simulink model "DynamicsPID_CompleteTest"  (R2018b)
settings: Solver=ode5  StartTime=0.0  StopTime=10  FixedStep=0.0001  RelTol=1e-3
PreLoadFcn:
  | load('Arm6SimscapeData.mat');
model workspace: external: MAT-File E:\SixRobotArm\Simscape_Simulation\Arm6SimscapeData.mat (data not in the file)
values from neighbouring files (symbols this model uses):
  smiData =     [Arm6SimscapeData.mat]
undefined symbols (not defined in the file or in its folder): X, Y, Z
libraries: sm_lib x36, nesl_utility x31, fl_lib x13, simulink x6
(part 1 of 2)
settings Model: SimulationMode=accelerator  Creator=Administrator  LastModifiedBy=Jeason
settings SolverCC: AutoInsertRateTranBlk=on
settings DataIOCC: ReturnWorkspaceOutputs=on
settings ExplorerConfigSet: InternalSimMechanicsExplorerSettings="<ExplorerConfiguration><canonicalview>planar_xy</canonicalview><AnimationSetting><BasePlaybackSpeed>1.0</BasePlaybackSpeed><PlaybackSpeedFactor>1.0</PlaybackSpeedFactor></AnimationSetting><TilePanel><TileInfo><Tiles Columns=\"1\" Count=\"1\" Rows=\"1\"><Column Weight=\"1\"/><Row Weight=\"1\"/><Tile Height=\"1\" Width=\"1\" X=\"0\" Y=\"0\"/></Tiles></TileInfo><SceneInfo><SceneViewer><BGColor><R>0.60000002384185791</R><G>0.60000002384185791</G><B>0.60000002384185791</B></BGColor><Camera><DoPerspective>off</DoPerspective><Position><X>0.529425685588477024</X><Y>0.96968881474758839</Y><Z>0.531520526083879341</Z></Position><Center><X>-0.0479245836011489429</X><Y>0.392338545557962604</Y><Z>-0.0458297431057466537</Z></Center><Up><X>-0.408248290463863073</X><Y>0.816496580927726145</Y><Z>-0.408248290463863073</Z></Up><ViewLimDist>1</ViewLimDist><YLim>0.78131541566616991</YLim><XLim>0.557104420151891211</XLim></Camera></SceneViewer></SceneInfo></TilePanel><MechEditorPanel><Cameras/><GfxPanelCameraMap/><VideoCreator><PlaybackSpeedRatio>1.0</PlaybackSpeedRatio><FrameRate>30</FrameRate><VideoFormat>MPEG-4</VideoFormat><FrameSize>[400 400]</FrameSize></VideoCreator></MechEditorPanel></ExplorerConfiguration>"

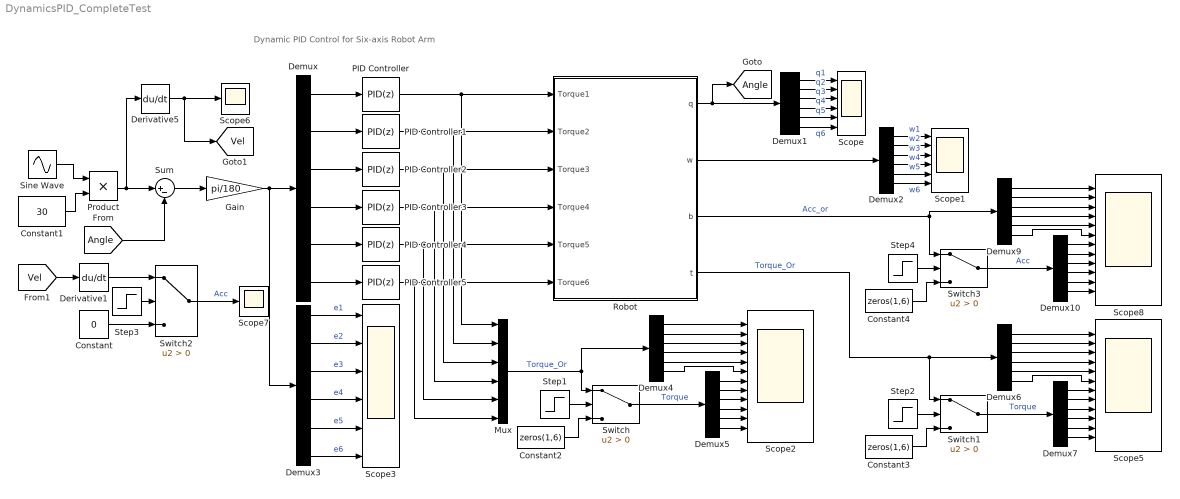
== system DynamicsPID_CompleteTest ==
  note: Dynamic PID Control for Six-axis Robot Arm
  Constant : Constant  Value=0
  Constant1 : Constant  Value=30
  Constant2 : Constant  Value=zeros(1,6)
  Constant3 : Constant  Value=zeros(1,6)
  Constant4 : Constant  Value=zeros(1,6)
  Demux{,1..7,9..10} (10 alike) : Demux  Outputs=6
  Derivative1 : Derivative
  Derivative5 : Derivative
  Gain : Gain  Gain=pi/180
  Mux : Mux  Inputs=6
  PID Controller : simulink/Continuous/PID Controller  Controller=PID  Form=Parallel  TimeDomain=Discrete-time  SampleTime=-1  IntegratorMethod=Forward Euler  FilterMethod=Forward Euler  ControllerParametersSource=internal  P=6578.50187258326  I=281577.896683485  D=27.3665494202085  UseFilter=on  N=17023.3251187192  TunerSelectOption=Transfer Function Based (PID Tuner App)  InitialConditionSource=internal  InitialConditionForIntegrator=0  InitialConditionForFilter=0  DifferentiatorICPrevScaledInput=0  ExternalReset=none  TrackingMode=off  Kt=1  LimitOutput=off  UpperSaturationLimit=inf  LowerSaturationLimit=-inf  LinearizeAsGain=on  AntiWindupMode=none  Kb=1  POutMin=[]  POutMax=[]  IOutMin=[]  IOutMax=[]  DOutMin=[]  DOutMax=[]  NOutMin=[]  NOutMax=[]  SumOutMin=[]  SumOutMax=[]  SaturationOutMin=[]  SaturationOutMax=[]  PParamMin=[]  PParamMax=[]  IParamMin=[]  IParamMax=[]  DParamMin=[]  DParamMax=[]  NParamMin=[]  NParamMax=[]  KbParamMin=[]  KbParamMax=[]  KtParamMin=[]  KtParamMax=[]  KbOutMin=[]  KbOutMax=[]  KtOutMin=[]  KtOutMax=[]  IntegratorOutMin=[]  IntegratorOutMax=[]  FilterOutMin=[]  FilterOutMax=[]  SumI1OutMin=[]  SumI1OutMax=[]  SumI2OutMin=[]  SumI2OutMax=[]  SumI3OutMin=[]  SumI3OutMax=[]  SumI4OutMin=[]  SumI4OutMax=[]  SumDOutMin=[]  SumDOutMax=[]  DifferentiatorOutMin=[]  DifferentiatorOutMax=[]  FilterDiffOutCoefMin=[]  FilterDiffOutCoefMax=[]  ReciprocalOutMin=[]  ReciprocalOutMax=[]  SumDenOutMin=[]  SumDenOutMax=[]  SumNumOutMin=[]  SumNumOutMax=[]  DivideOutMin=[]  DivideOutMax=[]  IntegratorContinuousStateAttributes=''  IntegratorStateMustResolveToSignalObject=off  IntegratorRTWStateStorageClass=Auto  FilterContinuousStateAttributes=''  FilterStateMustResolveToSignalObject=off  FilterRTWStateStorageClass=Auto  ParallelPVariant=InternalParameters  IdealPVariant=Disabled  IVariant=InternalParameters  DVariant=InternalParameters  IntegratorVariant=Discrete  SatVariant=Disabled  AWVariant=Passthrough  PCopyVariant=Disabled  TRVariant=Disabled  FdbkBlocksVariant=Forward  IdealPFdbkVariant=Disabled  SatFdbkVariant=Disabled  DerivativeFilterVariant=ForwardEulerFilter  NVariant=InternalParameters  NCopyVariant=Disabled  FilterICVariant=InternalICsFilter  IntegratorICVariant=InternalICs  ExternalResetVariant=Disabled  TRSumVariant=Passthrough  SumFdbkVariant=Disabled  SumVariant=Sum_PID
  PID Controller1 : simulink/Continuous/PID Controller  Controller=PID  Form=Parallel  TimeDomain=Discrete-time  SampleTime=-1  IntegratorMethod=Forward Euler  FilterMethod=Forward Euler  ControllerParametersSource=internal  P=10668.8664662437  I=445184.60715373  D=63.0054233348583  UseFilter=on  N=6162.16152893693  TunerSelectOption=Transfer Function Based (PID Tuner App)  InitialConditionSource=internal  InitialConditionForIntegrator=0  InitialConditionForFilter=0  DifferentiatorICPrevScaledInput=0  ExternalReset=none  TrackingMode=off  Kt=1  LimitOutput=off  UpperSaturationLimit=inf  LowerSaturationLimit=-inf  LinearizeAsGain=on  AntiWindupMode=none  Kb=1  POutMin=[]  POutMax=[]  IOutMin=[]  IOutMax=[]  DOutMin=[]  DOutMax=[]  NOutMin=[]  NOutMax=[]  SumOutMin=[]  SumOutMax=[]  SaturationOutMin=[]  SaturationOutMax=[]  PParamMin=[]  PParamMax=[]  IParamMin=[]  IParamMax=[]  DParamMin=[]  DParamMax=[]  NParamMin=[]  NParamMax=[]  KbParamMin=[]  KbParamMax=[]  KtParamMin=[]  KtParamMax=[]  KbOutMin=[]  KbOutMax=[]  KtOutMin=[]  KtOutMax=[]  IntegratorOutMin=[]  IntegratorOutMax=[]  FilterOutMin=[]  FilterOutMax=[]  SumI1OutMin=[]  SumI1OutMax=[]  SumI2OutMin=[]  SumI2OutMax=[]  SumI3OutMin=[]  SumI3OutMax=[]  SumI4OutMin=[]  SumI4OutMax=[]  SumDOutMin=[]  SumDOutMax=[]  DifferentiatorOutMin=[]  DifferentiatorOutMax=[]  FilterDiffOutCoefMin=[]  FilterDiffOutCoefMax=[]  ReciprocalOutMin=[]  ReciprocalOutMax=[]  SumDenOutMin=[]  SumDenOutMax=[]  SumNumOutMin=[]  SumNumOutMax=[]  DivideOutMin=[]  DivideOutMax=[]  IntegratorContinuousStateAttributes=''  IntegratorStateMustResolveToSignalObject=off  IntegratorRTWStateStorageClass=Auto  FilterContinuousStateAttributes=''  FilterStateMustResolveToSignalObject=off  FilterRTWStateStorageClass=Auto  ParallelPVariant=InternalParameters  IdealPVariant=Disabled  IVariant=InternalParameters  DVariant=InternalParameters  IntegratorVariant=Discrete  SatVariant=Disabled  AWVariant=Passthrough  PCopyVariant=Disabled  TRVariant=Disabled  FdbkBlocksVariant=Forward  IdealPFdbkVariant=Disabled  SatFdbkVariant=Disabled  DerivativeFilterVariant=ForwardEulerFilter  NVariant=InternalParameters  NCopyVariant=Disabled  FilterICVariant=InternalICsFilter  IntegratorICVariant=InternalICs  ExternalResetVariant=Disabled  TRSumVariant=Passthrough  SumFdbkVariant=Disabled  SumVariant=Sum_PID
  PID Controller2 : simulink/Continuous/PID Controller  Controller=PID  Form=Parallel  TimeDomain=Discrete-time  SampleTime=-1  IntegratorMethod=Forward Euler  FilterMethod=Forward Euler  ControllerParametersSource=internal  P=13614.8176617989  I=1609883.93215342  D=16.7397300352701  UseFilter=on  N=18647.3427476524  TunerSelectOption=Transfer Function Based (PID Tuner App)  InitialConditionSource=internal  InitialConditionForIntegrator=0  InitialConditionForFilter=0  DifferentiatorICPrevScaledInput=0  ExternalReset=none  TrackingMode=off  Kt=1  LimitOutput=off  UpperSaturationLimit=inf  LowerSaturationLimit=-inf  LinearizeAsGain=on  AntiWindupMode=none  Kb=1  POutMin=[]  POutMax=[]  IOutMin=[]  IOutMax=[]  DOutMin=[]  DOutMax=[]  NOutMin=[]  NOutMax=[]  SumOutMin=[]  SumOutMax=[]  SaturationOutMin=[]  SaturationOutMax=[]  PParamMin=[]  PParamMax=[]  IParamMin=[]  IParamMax=[]  DParamMin=[]  DParamMax=[]  NParamMin=[]  NParamMax=[]  KbParamMin=[]  KbParamMax=[]  KtParamMin=[]  KtParamMax=[]  KbOutMin=[]  KbOutMax=[]  KtOutMin=[]  KtOutMax=[]  IntegratorOutMin=[]  IntegratorOutMax=[]  FilterOutMin=[]  FilterOutMax=[]  SumI1OutMin=[]  SumI1OutMax=[]  SumI2OutMin=[]  SumI2OutMax=[]  SumI3OutMin=[]  SumI3OutMax=[]  SumI4OutMin=[]  SumI4OutMax=[]  SumDOutMin=[]  SumDOutMax=[]  DifferentiatorOutMin=[]  DifferentiatorOutMax=[]  FilterDiffOutCoefMin=[]  FilterDiffOutCoefMax=[]  ReciprocalOutMin=[]  ReciprocalOutMax=[]  SumDenOutMin=[]  SumDenOutMax=[]  SumNumOutMin=[]  SumNumOutMax=[]  DivideOutMin=[]  DivideOutMax=[]  IntegratorContinuousStateAttributes=''  IntegratorStateMustResolveToSignalObject=off  IntegratorRTWStateStorageClass=Auto  FilterContinuousStateAttributes=''  FilterStateMustResolveToSignalObject=off  FilterRTWStateStorageClass=Auto  ParallelPVariant=InternalParameters  IdealPVariant=Disabled  IVariant=InternalParameters  DVariant=InternalParameters  IntegratorVariant=Discrete  SatVariant=Disabled  AWVariant=Passthrough  PCopyVariant=Disabled  TRVariant=Disabled  FdbkBlocksVariant=Forward  IdealPFdbkVariant=Disabled  SatFdbkVariant=Disabled  DerivativeFilterVariant=ForwardEulerFilter  NVariant=InternalParameters  NCopyVariant=Disabled  FilterICVariant=InternalICsFilter  IntegratorICVariant=InternalICs  ExternalResetVariant=Disabled  TRSumVariant=Passthrough  SumFdbkVariant=Disabled  SumVariant=Sum_PID
  PID Controller3 : simulink/Continuous/PID Controller  Controller=PID  Form=Parallel  TimeDomain=Discrete-time  SampleTime=-1  IntegratorMethod=Forward Euler  FilterMethod=Forward Euler  ControllerParametersSource=internal  P=2278.44727281027  I=57632.5068461777  D=4.78900982736188  UseFilter=on  N=12334.3834454525  TunerSelectOption=Transfer Function Based (PID Tuner App)  InitialConditionSource=internal  InitialConditionForIntegrator=0  InitialConditionForFilter=0  DifferentiatorICPrevScaledInput=0  ExternalReset=none  TrackingMode=off  Kt=1  LimitOutput=off  UpperSaturationLimit=inf  LowerSaturationLimit=-inf  LinearizeAsGain=on  AntiWindupMode=none  Kb=1  POutMin=[]  POutMax=[]  IOutMin=[]  IOutMax=[]  DOutMin=[]  DOutMax=[]  NOutMin=[]  NOutMax=[]  SumOutMin=[]  SumOutMax=[]  SaturationOutMin=[]  SaturationOutMax=[]  PParamMin=[]  PParamMax=[]  IParamMin=[]  IParamMax=[]  DParamMin=[]  DParamMax=[]  NParamMin=[]  NParamMax=[]  KbParamMin=[]  KbParamMax=[]  KtParamMin=[]  KtParamMax=[]  KbOutMin=[]  KbOutMax=[]  KtOutMin=[]  KtOutMax=[]  IntegratorOutMin=[]  IntegratorOutMax=[]  FilterOutMin=[]  FilterOutMax=[]  SumI1OutMin=[]  SumI1OutMax=[]  SumI2OutMin=[]  SumI2OutMax=[]  SumI3OutMin=[]  SumI3OutMax=[]  SumI4OutMin=[]  SumI4OutMax=[]  SumDOutMin=[]  SumDOutMax=[]  DifferentiatorOutMin=[]  DifferentiatorOutMax=[]  FilterDiffOutCoefMin=[]  FilterDiffOutCoefMax=[]  ReciprocalOutMin=[]  ReciprocalOutMax=[]  SumDenOutMin=[]  SumDenOutMax=[]  SumNumOutMin=[]  SumNumOutMax=[]  DivideOutMin=[]  DivideOutMax=[]  IntegratorContinuousStateAttributes=''  IntegratorStateMustResolveToSignalObject=off  IntegratorRTWStateStorageClass=Auto  FilterContinuousStateAttributes=''  FilterStateMustResolveToSignalObject=off  FilterRTWStateStorageClass=Auto  ParallelPVariant=InternalParameters  IdealPVariant=Disabled  IVariant=InternalParameters  DVariant=InternalParameters  IntegratorVariant=Discrete  SatVariant=Disabled  AWVariant=Passthrough  PCopyVariant=Disabled  TRVariant=Disabled  FdbkBlocksVariant=Forward  IdealPFdbkVariant=Disabled  SatFdbkVariant=Disabled  DerivativeFilterVariant=ForwardEulerFilter  NVariant=InternalParameters  NCopyVariant=Disabled  FilterICVariant=InternalICsFilter  IntegratorICVariant=InternalICs  ExternalResetVariant=Disabled  TRSumVariant=Passthrough  SumFdbkVariant=Disabled  SumVariant=Sum_PID
  PID Controller4 : simulink/Continuous/PID Controller  Controller=PID  Form=Parallel  TimeDomain=Discrete-time  SampleTime=-1  IntegratorMethod=Forward Euler  FilterMethod=Forward Euler  ControllerParametersSource=internal  P=162.012170441032  I=2991.2299773876  D=1.94609590633376  UseFilter=on  N=18952.9125503668  TunerSelectOption=Transfer Function Based (PID Tuner App)  InitialConditionSource=internal  InitialConditionForIntegrator=0  InitialConditionForFilter=0  DifferentiatorICPrevScaledInput=0  ExternalReset=none  TrackingMode=off  Kt=1  LimitOutput=off  UpperSaturationLimit=inf  LowerSaturationLimit=-inf  LinearizeAsGain=on  AntiWindupMode=none  Kb=1  POutMin=[]  POutMax=[]  IOutMin=[]  IOutMax=[]  DOutMin=[]  DOutMax=[]  NOutMin=[]  NOutMax=[]  SumOutMin=[]  SumOutMax=[]  SaturationOutMin=[]  SaturationOutMax=[]  PParamMin=[]  PParamMax=[]  IParamMin=[]  IParamMax=[]  DParamMin=[]  DParamMax=[]  NParamMin=[]  NParamMax=[]  KbParamMin=[]  KbParamMax=[]  KtParamMin=[]  KtParamMax=[]  KbOutMin=[]  KbOutMax=[]  KtOutMin=[]  KtOutMax=[]  IntegratorOutMin=[]  IntegratorOutMax=[]  FilterOutMin=[]  FilterOutMax=[]  SumI1OutMin=[]  SumI1OutMax=[]  SumI2OutMin=[]  SumI2OutMax=[]  SumI3OutMin=[]  SumI3OutMax=[]  SumI4OutMin=[]  SumI4OutMax=[]  SumDOutMin=[]  SumDOutMax=[]  DifferentiatorOutMin=[]  DifferentiatorOutMax=[]  FilterDiffOutCoefMin=[]  FilterDiffOutCoefMax=[]  ReciprocalOutMin=[]  ReciprocalOutMax=[]  SumDenOutMin=[]  SumDenOutMax=[]  SumNumOutMin=[]  SumNumOutMax=[]  DivideOutMin=[]  DivideOutMax=[]  IntegratorContinuousStateAttributes=''  IntegratorStateMustResolveToSignalObject=off  IntegratorRTWStateStorageClass=Auto  FilterContinuousStateAttributes=''  FilterStateMustResolveToSignalObject=off  FilterRTWStateStorageClass=Auto  ParallelPVariant=InternalParameters  IdealPVariant=Disabled  IVariant=InternalParameters  DVariant=InternalParameters  IntegratorVariant=Discrete  SatVariant=Disabled  AWVariant=Passthrough  PCopyVariant=Disabled  TRVariant=Disabled  FdbkBlocksVariant=Forward  IdealPFdbkVariant=Disabled  SatFdbkVariant=Disabled  DerivativeFilterVariant=ForwardEulerFilter  NVariant=InternalParameters  NCopyVariant=Disabled  FilterICVariant=InternalICsFilter  IntegratorICVariant=InternalICs  ExternalResetVariant=Disabled  TRSumVariant=Passthrough  SumFdbkVariant=Disabled  SumVariant=Sum_PID
  PID Controller5 : simulink/Continuous/PID Controller  Controller=PID  Form=Parallel  TimeDomain=Discrete-time  SampleTime=-1  IntegratorMethod=Forward Euler  FilterMethod=Forward Euler  ControllerParametersSource=internal  P=53.1250888383144  I=2127.20939788441  D=0.32148544609688  UseFilter=on  N=3458.79738025908  TunerSelectOption=Transfer Function Based (PID Tuner App)  InitialConditionSource=internal  InitialConditionForIntegrator=0  InitialConditionForFilter=0  DifferentiatorICPrevScaledInput=0  ExternalReset=none  TrackingMode=off  Kt=1  LimitOutput=off  UpperSaturationLimit=inf  LowerSaturationLimit=-inf  LinearizeAsGain=on  AntiWindupMode=none  Kb=1  POutMin=[]  POutMax=[]  IOutMin=[]  IOutMax=[]  DOutMin=[]  DOutMax=[]  NOutMin=[]  NOutMax=[]  SumOutMin=[]  SumOutMax=[]  SaturationOutMin=[]  SaturationOutMax=[]  PParamMin=[]  PParamMax=[]  IParamMin=[]  IParamMax=[]  DParamMin=[]  DParamMax=[]  NParamMin=[]  NParamMax=[]  KbParamMin=[]  KbParamMax=[]  KtParamMin=[]  KtParamMax=[]  KbOutMin=[]  KbOutMax=[]  KtOutMin=[]  KtOutMax=[]  IntegratorOutMin=[]  IntegratorOutMax=[]  FilterOutMin=[]  FilterOutMax=[]  SumI1OutMin=[]  SumI1OutMax=[]  SumI2OutMin=[]  SumI2OutMax=[]  SumI3OutMin=[]  SumI3OutMax=[]  SumI4OutMin=[]  SumI4OutMax=[]  SumDOutMin=[]  SumDOutMax=[]  DifferentiatorOutMin=[]  DifferentiatorOutMax=[]  FilterDiffOutCoefMin=[]  FilterDiffOutCoefMax=[]  ReciprocalOutMin=[]  ReciprocalOutMax=[]  SumDenOutMin=[]  SumDenOutMax=[]  SumNumOutMin=[]  SumNumOutMax=[]  DivideOutMin=[]  DivideOutMax=[]  IntegratorContinuousStateAttributes=''  IntegratorStateMustResolveToSignalObject=off  IntegratorRTWStateStorageClass=Auto  FilterContinuousStateAttributes=''  FilterStateMustResolveToSignalObject=off  FilterRTWStateStorageClass=Auto  ParallelPVariant=InternalParameters  IdealPVariant=Disabled  IVariant=InternalParameters  DVariant=InternalParameters  IntegratorVariant=Discrete  SatVariant=Disabled  AWVariant=Passthrough  PCopyVariant=Disabled  TRVariant=Disabled  FdbkBlocksVariant=Forward  IdealPFdbkVariant=Disabled  SatFdbkVariant=Disabled  DerivativeFilterVariant=ForwardEulerFilter  NVariant=InternalParameters  NCopyVariant=Disabled  FilterICVariant=InternalICsFilter  IntegratorICVariant=InternalICs  ExternalResetVariant=Disabled  TRSumVariant=Passthrough  SumFdbkVariant=Disabled  SumVariant=Sum_PID
  Product : Product
  Robot : Subsystem
  Scope : Scope  NumInputPorts=6
  Scope1 : Scope  NumInputPorts=6
  Scope2 : Scope  NumInputPorts=12
  Scope3 : Scope  NumInputPorts=6
  Scope5 : Scope  NumInputPorts=12
  Scope6 : Scope
  Scope7 : Scope
  Scope8 : Scope  NumInputPorts=12
  Sine Wave : Sin  Frequency=0.25*2*pi
  Step1 : Step  Time=0.3  After=2
  Step2 : Step  Time=0.1  After=2
  Step3 : Step  Time=0.1  After=2
  Step4 : Step  Time=0.3  After=2
  Sum : Sum  Inputs=|+-
  Switch{,1..3} (4 alike) : Switch  Criteria=u2 > Threshold
  tag scope: Angle=global, Vel=global
  wires:
  Robot/1(q) -> Demux1/1, [Angle]
  Demux1/1 -> Scope/1  "q1"
  Demux1/2 -> Scope/2  "q2"
  Demux1/3 -> Scope/3  "q3"
  Demux1/4 -> Scope/4  "q4"
  Demux1/5 -> Scope/5  "q5"
  Demux1/6 -> Scope/6  "q6"
  Robot/2(w) -> Demux2/1
  Demux2/1 -> Scope1/1  "w1"
  Demux2/2 -> Scope1/2  "w2"
  Demux2/3 -> Scope1/3  "w3"
  Demux2/4 -> Scope1/4  "w4"
  Demux2/5 -> Scope1/5  "w5"
  Demux2/6 -> Scope1/6  "w6"
  Constant1/1 -> Product/2
  Sine Wave/1 -> Product/1
  Constant2/1 -> Switch/3
  Step1/1 -> Switch/2
  Mux/1 -> Switch/1, Demux4/1  "Torque_Or"
  Sum/1 -> Gain/1
  [Angle] -> Sum/2
  Gain/1 -> Demux3/1, Demux/1
  Demux/1 -> PID Controller/1
  Demux/2 -> PID Controller1/1
  Demux/3 -> PID Controller2/1
  Demux/4 -> PID Controller3/1
  Demux/5 -> PID Controller4/1
  Demux/6 -> PID Controller5/1
  PID Controller/1 -> Robot/1(Torque1), Mux/1
  PID Controller1/1 -> Robot/2(Torque2), Mux/2
  PID Controller2/1 -> Robot/3(Torque3), Mux/3
  PID Controller3/1 -> Robot/4(Torque4), Mux/4
  PID Controller4/1 -> Robot/5(Torque5), Mux/5
  PID Controller5/1 -> Robot/6(Torque6), Mux/6
  Demux3/1 -> Scope3/1  "e1"
  Demux3/2 -> Scope3/2  "e2"
  Demux3/3 -> Scope3/3  "e3"
  Demux3/4 -> Scope3/4  "e4"
  Demux3/5 -> Scope3/5  "e5"
  Demux3/6 -> Scope3/6  "e6"
  Demux4/2 -> Scope2/2
  Demux4/1 -> Scope2/1
  Demux4/3 -> Scope2/3
  Demux4/4 -> Scope2/4
  Demux4/5 -> Scope2/5
  Demux4/6 -> Scope2/6
  Demux5/2 -> Scope2/8
  Demux5/1 -> Scope2/7
  Demux5/3 -> Scope2/9
  Demux5/4 -> Scope2/10
  Demux5/5 -> Scope2/11
  Demux5/6 -> Scope2/12
  Switch/1 -> Demux5/1  "Torque"
  Switch1/1 -> Demux7/1  "Torque"
  Demux7/6 -> Scope5/12
  Demux7/5 -> Scope5/11
  Demux7/4 -> Scope5/10
  Demux7/3 -> Scope5/9
  Demux7/1 -> Scope5/7
  Demux7/2 -> Scope5/8
  Demux6/6 -> Scope5/6
  Demux6/5 -> Scope5/5
  Demux6/4 -> Scope5/4
  Demux6/3 -> Scope5/3
  Demux6/1 -> Scope5/1
  Demux6/2 -> Scope5/2
  Robot/4(t) -> Switch1/1, Demux6/1  "Torque_Or"
  Step2/1 -> Switch1/2
  Constant3/1 -> Switch1/3
  Product/1 -> Sum/1, Derivative5/1
  Derivative5/1 -> [Vel], Scope6/1
  Derivative1/1 -> Switch2/1
  Step3/1 -> Switch2/2
  [Vel] -> Derivative1/1
  Constant/1 -> Switch2/3
  Switch2/1 -> Scope7/1  "Acc"
  Constant4/1 -> Switch3/3
  Step4/1 -> Switch3/2
  Robot/3(b) -> Demux9/1, Switch3/1  "Acc_or"
  Demux9/2 -> Scope8/2
  Demux9/1 -> Scope8/1
  Demux9/3 -> Scope8/3
  Demux9/4 -> Scope8/4
  Demux9/5 -> Scope8/5
  Demux9/6 -> Scope8/6
  Demux10/2 -> Scope8/8
  Demux10/1 -> Scope8/7
  Demux10/3 -> Scope8/9
  Demux10/4 -> Scope8/10
  Demux10/5 -> Scope8/11
  Demux10/6 -> Scope8/12
  Switch3/1 -> Demux10/1  "Acc"

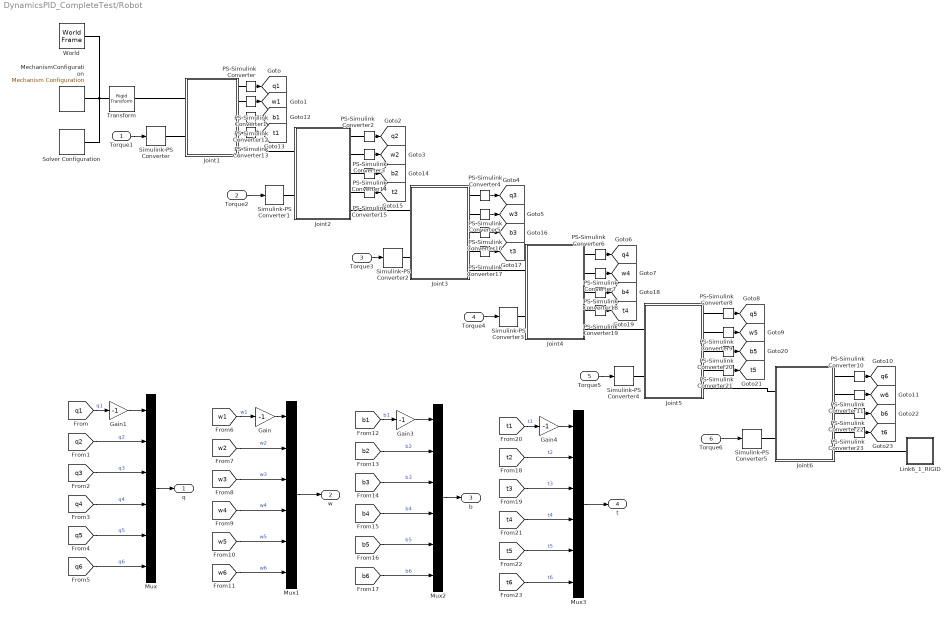
== system DynamicsPID_CompleteTest/Robot ==
  Torque1 : Inport
  Torque2 : Inport  Port=2
  Torque3 : Inport  Port=3
  Torque4 : Inport  Port=4
  Torque5 : Inport  Port=5
  Torque6 : Inport  Port=6
  Gain{,1,3..4} (4 alike) : Gain  Gain=-1
  Joint1 : Subsystem
  Joint2 : Subsystem
  Joint3 : Subsystem
  Joint4 : Subsystem
  Joint5 : Subsystem
  Joint6 : Subsystem
  Link6_1_RIGID : Subsystem
  MechanismConfiguration : sm_lib/Utilities/Mechanism Configuration  UniformGravity=Constant  GravityVector=[0 -9.80665 0]  GravityUnits=m/s^2  LinearizationDelta=0.001
  Mux{,1..3} (4 alike) : Mux  Inputs=6
  PS-Simulink Converter{,2,4,6,8,10} (6 alike) : nesl_utility/PS-Simulink Converter  PhysicalDomain=network_engine_domain  SubClassName=ps_output  LeftPortType=input  RightPortType=output  PseudoPeriodic=off  Frequencies=[]  Unit=deg  AffineConversion=off
  PS-Simulink Converter{1,3,5,7,9,11} (6 alike) : nesl_utility/PS-Simulink Converter  PhysicalDomain=network_engine_domain  SubClassName=ps_output  LeftPortType=input  RightPortType=output  PseudoPeriodic=off  Frequencies=[]  Unit=deg/s  AffineConversion=off
  PS-Simulink Converter{12,14,16,18,20,22} (6 alike) : nesl_utility/PS-Simulink Converter  PhysicalDomain=network_engine_domain  SubClassName=ps_output  LeftPortType=input  RightPortType=output  PseudoPeriodic=off  Frequencies=[]  Unit=deg/s^2  AffineConversion=off
  PS-Simulink Converter{13,15,17,19,21,23} (6 alike) : nesl_utility/PS-Simulink Converter  PhysicalDomain=network_engine_domain  SubClassName=ps_output  LeftPortType=input  RightPortType=output  PseudoPeriodic=off  Frequencies=[]  Unit=N*m  AffineConversion=off
  Simulink-PS Converter{,1..5} (6 alike) : nesl_utility/Simulink-PS Converter  PhysicalDomain=network_engine_domain  SubClassName=ps_input  LeftPortType=input  RightPortType=output  PseudoPeriodic=off  Frequencies=[]  NoiseDistribution=none  NoiseParameters=[]  Unit=N*m  AffineConversion=off  FilteringAndDerivatives=provide  SimscapeFilterOrder=2  InputFilterTimeConstant=0.001  UdotUserProvided=0
  Solver Configuration : nesl_utility/Solver Configuration  PhysicalDomain=network_engine_domain  SubClassName=solver  LeftPortType=input  RightPortType=generic  Tones=[]  Harmonics=[]  SimulateNoise=off  Profile=off  UseLocalSampling=off  EnableSwitchedLinearOptims=on  FrequencyDomain=off  UseCCode=off  RelTol=0.001  AbsTol=1e-06  MinStep=1e-09  ToWorkspace=off  RevertToSquareIcSolve=off  NumHomotopyIterations=100  PhasorMode=off  PhasorModeNumHarmonics=1  DoDC=off  ResidualTolerance=1e-09  UseLocalSolver=off  LocalSolverChoice=NE_BACKWARD_EULER_ADVANCER  LocalSolverSampleTime=0.001  DoFixedCost=off  MaxNonlinIter=3  MaxModeIter=2  LinearAlgebra=auto  EquationFormulation=NE_TIME_EF  DelaysMemoryBudget=1024  AutomaticFiltering=on  FilteringTimeConstant=0.001  PartitionStorageMethod=AS_NEEDED  PartitionMemoryBudget=1024
  Transform : sm_lib/Frames and Transforms/Rigid Transform  TranslationMethod=Cartesian  TranslationStandardOffset=0  TranslationLengthUnit=mm  TranslationStandardAxis=+Z  TranslationCartesianOffset=smiData.RigidTransform(14).translation  TranslationROffset=0  TranslationROffsetUnits=m  TranslationZOffset=0  TranslationZOffsetUnits=m  TranslationThetaOffset=0  TranslationThetaOffsetUnits=deg  RotationMethod=ArbitraryAxis  RotationAngleUnits=rad  RotationStandardAxis=+Z  RotationAngle=smiData.RigidTransform(14).angle  RotationArbitraryAxis=smiData.RigidTransform(14).axis  FollAlignAxisA=+X  BaseAlignAxisA=+Y  FollAlignAxisB=+Y  BaseAlignAxisB=+Z  RotationSequenceAxes=FollowerAxes  RotationSequence=XYX  RotationSequenceAngles=[0 0 0]  RotationSequenceAnglesUnits=deg  RotationMatrix=[1 0 0; 0 1 0; 0 0 1]
  World : sm_lib/Frames and Transforms/World Frame
  q : Outport  VectorParamsAs1DForOutWhenUnconnected=on
  w : Outport  Port=2  VectorParamsAs1DForOutWhenUnconnected=on
  b : Outport  Port=3  VectorParamsAs1DForOutWhenUnconnected=on
  t : Outport  Port=4  VectorParamsAs1DForOutWhenUnconnected=on
  tag scope: b1=global, b2=global, b3=global, b4=global, b5=global, b6=global, q1=global, q2=global, q3=global, q4=global, q5=global, q6=global, t1=global, t2=global, t3=global, t4=global, t5=global, t6=global, w1=global, w2=global, w3=global, w4=global, w5=global, w6=global
  wires:
  [q5] -> Mux/5  "q5"
  Mux/1 -> q/1
  PS-Simulink Converter6/1 -> [q4]
  [w4] -> Mux1/4  "w4"
  PS-Simulink Converter/1 -> [q1]
  [q6] -> Mux/6  "q6"
  [w1] -> Gain/1  "w1"
  [w5] -> Mux1/5  "w5"
  PS-Simulink Converter4/1 -> [q3]
  PS-Simulink Converter5/1 -> [w3]
  PS-Simulink Converter9/1 -> [w5]
  [w2] -> Mux1/2  "w2"
  PS-Simulink Converter1/1 -> [w1]
  [q2] -> Mux/2  "q2"
  PS-Simulink Converter10/1 -> [q6]
  [w6] -> Mux1/6  "w6"
  PS-Simulink Converter7/1 -> [w4]
  [q4] -> Mux/4  "q4"
  PS-Simulink Converter11/1 -> [w6]
  PS-Simulink Converter8/1 -> [q5]
  Mux1/1 -> w/1
  PS-Simulink Converter2/1 -> [q2]
  [q3] -> Mux/3  "q3"
  [q1] -> Gain1/1  "q1"
  [w3] -> Mux1/3  "w3"
  PS-Simulink Converter3/1 -> [w2]
  Torque2/1 -> Simulink-PS Converter1/1
  Torque3/1 -> Simulink-PS Converter2/1
  Torque4/1 -> Simulink-PS Converter3/1
  Torque5/1 -> Simulink-PS Converter4/1
  Torque6/1 -> Simulink-PS Converter5/1
  Gain/1 -> Mux1/1
  Gain1/1 -> Mux/1
  PS-Simulink Converter12/1 -> [b1]
  PS-Simulink Converter13/1 -> [t1]
  PS-Simulink Converter15/1 -> [t2]
  PS-Simulink Converter14/1 -> [b2]
  PS-Simulink Converter16/1 -> [b3]
  PS-Simulink Converter17/1 -> [t3]
  PS-Simulink Converter19/1 -> [t4]
  PS-Simulink Converter18/1 -> [b4]
  PS-Simulink Converter20/1 -> [b5]
  PS-Simulink Converter21/1 -> [t5]
  PS-Simulink Converter23/1 -> [t6]
  PS-Simulink Converter22/1 -> [b6]
  Gain3/1 -> Mux2/1
  [b1] -> Gain3/1  "b1"
  Mux3/1 -> t/1
  [t1] -> Gain4/1  "t1"
  Mux2/1 -> b/1
  [b2] -> Mux2/2  "b2"
  [b3] -> Mux2/3  "b3"
  [b4] -> Mux2/4  "b4"
  [b5] -> Mux2/5  "b5"
  [b6] -> Mux2/6  "b6"
  [t2] -> Mux3/2  "t2"
  [t3] -> Mux3/3  "t3"
  [t4] -> Mux3/4  "t4"
  [t5] -> Mux3/5  "t5"
  [t6] -> Mux3/6  "t6"
  Torque1/1 -> Simulink-PS Converter/1
  Gain4/1 -> Mux3/1
  connections:
  Joint6/RConn1 -- PS-Simulink Converter10/LConn1
  PS-Simulink Converter11/LConn1 -- Joint6/RConn2
  Joint4/RConn2 -- PS-Simulink Converter7/LConn1
  Joint4/RConn1 -- PS-Simulink Converter6/LConn1
  PS-Simulink Converter9/LConn1 -- Joint5/RConn2
  PS-Simulink Converter5/LConn1 -- Joint3/RConn2
  Transform/LConn1 -- MechanismConfiguration/RConn1 -- Solver Configuration/RConn1 -- World/RConn1
  Joint3/RConn5 -- Joint4/LConn1
  Joint1/RConn2 -- PS-Simulink Converter1/LConn1
  PS-Simulink Converter3/LConn1 -- Joint2/RConn2
  Joint1/LConn1 -- Transform/RConn1
  PS-Simulink Converter8/LConn1 -- Joint5/RConn1
  Simulink-PS Converter3/RConn1 -- Joint4/LConn2
  PS-Simulink Converter4/LConn1 -- Joint3/RConn1
  Joint1/RConn1 -- PS-Simulink Converter/LConn1
  Joint6/LConn1 -- Joint5/RConn5
  Joint3/LConn1 -- Joint2/RConn5
  Joint5/LConn1 -- Joint4/RConn5
  Link6_1_RIGID/LConn1 -- Joint6/RConn5
  Simulink-PS Converter5/RConn1 -- Joint6/LConn2
  Simulink-PS Converter1/RConn1 -- Joint2/LConn2
  PS-Simulink Converter2/LConn1 -- Joint2/RConn1
  Joint5/LConn2 -- Simulink-PS Converter4/RConn1
  Joint2/LConn1 -- Joint1/RConn5
  Simulink-PS Converter2/RConn1 -- Joint3/LConn2
  PS-Simulink Converter12/LConn1 -- Joint1/RConn3
  PS-Simulink Converter13/LConn1 -- Joint1/RConn4
  PS-Simulink Converter15/LConn1 -- Joint2/RConn4
  PS-Simulink Converter14/LConn1 -- Joint2/RConn3
  PS-Simulink Converter16/LConn1 -- Joint3/RConn3
  Joint3/RConn4 -- PS-Simulink Converter17/LConn1
  PS-Simulink Converter18/LConn1 -- Joint4/RConn3
  PS-Simulink Converter19/LConn1 -- Joint4/RConn4
  PS-Simulink Converter20/LConn1 -- Joint5/RConn3
  PS-Simulink Converter21/LConn1 -- Joint5/RConn4
  PS-Simulink Converter23/LConn1 -- Joint6/RConn4
  Joint6/RConn3 -- PS-Simulink Converter22/LConn1
  Joint1/LConn2 -- Simulink-PS Converter/RConn1

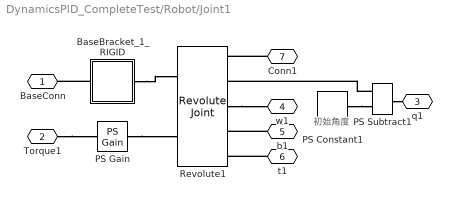
== system DynamicsPID_CompleteTest/Robot/Joint1 ==
  note: 初始角度
  BaseBracket_1_RIGID : Subsystem
  PS Constant1 : fl_lib/Physical Signals/Sources/PS Constant  constant=-pi/2
  PS Gain : fl_lib/Physical Signals/Functions/PS Gain  gain=-1
  PS Subtract1 : fl_lib/Physical Signals/Functions/PS Subtract
      settings: SourceProductName=Simscape
  Revolute1 : sm_lib/Joints/Revolute Joint  SenseConstraintForce=off  SenseConstraintForceX=off  SenseConstraintForceY=off  SenseConstraintForceZ=off  SenseConstraintTorque=off  SenseConstraintTorqueX=off  SenseConstraintTorqueY=off  SenseConstraintTorqueZ=off  SenseTotalForce=off  SenseTotalForceX=off  SenseTotalForceY=off  SenseTotalForceZ=off  SenseTotalTorque=off  SenseTotalTorqueX=off  SenseTotalTorqueY=off  SenseTotalTorqueZ=off  CompositeWrenchDir=FollowerOnBase  CompositeWrenchFrame=BaseFrame  EquilibriumPosition=0  EquilibriumPositionUnits=rad  SpringStiffness=0  SpringStiffnessUnits=N*m/rad  DampingCoefficient=0  DampingCoefficientUnits=N*m/(rad/s)  TorqueActuationMode=InputTorque  MotionActuationMode=ComputedMotion  SensePosition=on  SenseVelocity=on  SenseAcceleration=on  SenseTorqueForce=on  PositionTargetSpecify=on  PositionTargetPriority=Low  PositionTargetValue=smiData.RevoluteJoint(2).Rz.Pos  PositionTargetValueUnits=deg  VelocityTargetSpecify=off  VelocityTargetPriority=High  VelocityTargetValue=0  VelocityTargetValueUnits=deg/s
  BaseConn : PMIOPort  Side=Left
  Torque1 : PMIOPort  Port=2  Side=Left
  q1 : PMIOPort  Port=3  Side=Right
  w1 : PMIOPort  Port=4  Side=Right
  b1 : PMIOPort  Port=5  Side=Right
  t1 : PMIOPort  Port=6  Side=Right
  Conn1 : PMIOPort  Port=7  Side=Right
  connections:
  BaseBracket_1_RIGID/RConn1 -- Revolute1/LConn1
  Conn1/RConn1 -- Revolute1/RConn1
  BaseBracket_1_RIGID/LConn1 -- BaseConn/RConn1
  PS Subtract1/LConn1 -- Revolute1/RConn2
  PS Constant1/RConn1 -- PS Subtract1/LConn2
  PS Subtract1/RConn1 -- q1/RConn1
  Revolute1/RConn3 -- w1/RConn1
  Torque1/RConn1 -- PS Gain/LConn1
  b1/RConn1 -- Revolute1/RConn4
  t1/RConn1 -- Revolute1/RConn5
  PS Gain/RConn1 -- Revolute1/LConn2

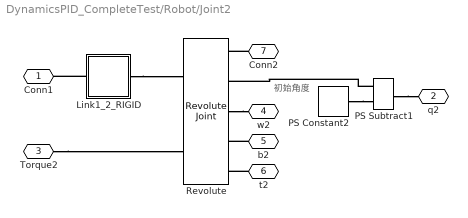
== system DynamicsPID_CompleteTest/Robot/Joint2 ==
  note: 初始角度
  Link1_2_RIGID : Subsystem
  PS Constant2 : fl_lib/Physical Signals/Sources/PS Constant  constant=-pi/2
  PS Subtract1 : fl_lib/Physical Signals/Functions/PS Subtract
      settings: SourceProductName=Simscape
  Revolute : sm_lib/Joints/Revolute Joint  SenseConstraintForce=off  SenseConstraintForceX=off  SenseConstraintForceY=off  SenseConstraintForceZ=off  SenseConstraintTorque=off  SenseConstraintTorqueX=off  SenseConstraintTorqueY=off  SenseConstraintTorqueZ=off  SenseTotalForce=off  SenseTotalForceX=off  SenseTotalForceY=off  SenseTotalForceZ=off  SenseTotalTorque=off  SenseTotalTorqueX=off  SenseTotalTorqueY=off  SenseTotalTorqueZ=off  CompositeWrenchDir=FollowerOnBase  CompositeWrenchFrame=BaseFrame  EquilibriumPosition=0  EquilibriumPositionUnits=rad  SpringStiffness=0  SpringStiffnessUnits=N*m/rad  DampingCoefficient=0  DampingCoefficientUnits=N*m/(rad/s)  TorqueActuationMode=InputTorque  MotionActuationMode=ComputedMotion  SensePosition=on  SenseVelocity=on  SenseAcceleration=on  SenseTorqueForce=on  PositionTargetSpecify=on  PositionTargetPriority=Low  PositionTargetValue=smiData.RevoluteJoint(1).Rz.Pos  PositionTargetValueUnits=deg  VelocityTargetSpecify=off  VelocityTargetPriority=High  VelocityTargetValue=0  VelocityTargetValueUnits=deg/s
  Conn1 : PMIOPort  Side=Left
  q2 : PMIOPort  Port=2  Side=Right
  Torque2 : PMIOPort  Port=3  Side=Left
  w2 : PMIOPort  Port=4  Side=Right
  b2 : PMIOPort  Port=5  Side=Right
  t2 : PMIOPort  Port=6  Side=Right
  Conn2 : PMIOPort  Port=7  Side=Right
  connections:
  Link1_2_RIGID/LConn1 -- Conn1/RConn1
  Link1_2_RIGID/RConn1 -- Revolute/LConn1
  Conn2/RConn1 -- Revolute/RConn1
  PS Subtract1/LConn1 -- Revolute/RConn2
  Revolute/RConn3 -- w2/RConn1
  Torque2/RConn1 -- Revolute/LConn2
  PS Constant2/RConn1 -- PS Subtract1/LConn2
  PS Subtract1/RConn1 -- q2/RConn1
  b2/RConn1 -- Revolute/RConn4
  t2/RConn1 -- Revolute/RConn5

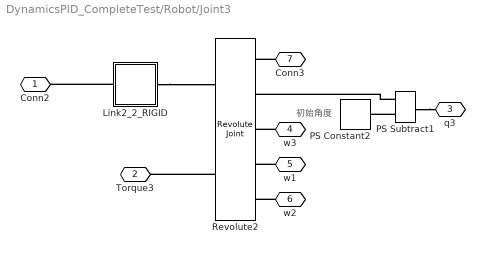
== system DynamicsPID_CompleteTest/Robot/Joint3 ==
  note: 初始角度
  Link2_2_RIGID : Subsystem
  PS Constant2 : fl_lib/Physical Signals/Sources/PS Constant  constant=0
  PS Subtract1 : fl_lib/Physical Signals/Functions/PS Subtract
      settings: SourceProductName=Simscape
  Revolute2 : sm_lib/Joints/Revolute Joint  SenseConstraintForce=off  SenseConstraintForceX=off  SenseConstraintForceY=off  SenseConstraintForceZ=off  SenseConstraintTorque=off  SenseConstraintTorqueX=off  SenseConstraintTorqueY=off  SenseConstraintTorqueZ=off  SenseTotalForce=off  SenseTotalForceX=off  SenseTotalForceY=off  SenseTotalForceZ=off  SenseTotalTorque=off  SenseTotalTorqueX=off  SenseTotalTorqueY=off  SenseTotalTorqueZ=off  CompositeWrenchDir=FollowerOnBase  CompositeWrenchFrame=BaseFrame  EquilibriumPosition=0  EquilibriumPositionUnits=rad  SpringStiffness=0  SpringStiffnessUnits=N*m/rad  DampingCoefficient=0  DampingCoefficientUnits=N*m/(rad/s)  TorqueActuationMode=InputTorque  MotionActuationMode=ComputedMotion  SensePosition=on  SenseVelocity=on  SenseAcceleration=on  SenseTorqueForce=on  PositionTargetSpecify=on  PositionTargetPriority=Low  PositionTargetValue=smiData.RevoluteJoint(3).Rz.Pos  PositionTargetValueUnits=deg  VelocityTargetSpecify=off  VelocityTargetPriority=High  VelocityTargetValue=0  VelocityTargetValueUnits=deg/s
  Conn2 : PMIOPort  Side=Left
  Torque3 : PMIOPort  Port=2  Side=Left
  q3 : PMIOPort  Port=3  Side=Right
  w3 : PMIOPort  Port=4  Side=Right
  w1 : PMIOPort  Port=5  Side=Right
  w2 : PMIOPort  Port=6  Side=Right
  Conn3 : PMIOPort  Port=7  Side=Right
  connections:
  Link2_2_RIGID/RConn1 -- Revolute2/LConn1
  Link2_2_RIGID/LConn1 -- Conn2/RConn1
  Revolute2/LConn2 -- Torque3/RConn1
  Conn3/RConn1 -- Revolute2/RConn1
  PS Subtract1/LConn2 -- PS Constant2/RConn1
  PS Subtract1/RConn1 -- q3/RConn1
  PS Subtract1/LConn1 -- Revolute2/RConn2
  w3/RConn1 -- Revolute2/RConn3
  w1/RConn1 -- Revolute2/RConn4
  w2/RConn1 -- Revolute2/RConn5

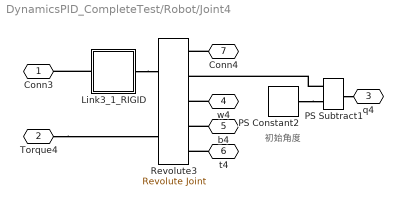
== system DynamicsPID_CompleteTest/Robot/Joint4 ==
  note: 初始角度
  Link3_1_RIGID : Subsystem
  PS Constant2 : fl_lib/Physical Signals/Sources/PS Constant  constant=0
  PS Subtract1 : fl_lib/Physical Signals/Functions/PS Subtract
      settings: SourceProductName=Simscape
  Revolute3 : sm_lib/Joints/Revolute Joint  SenseConstraintForce=off  SenseConstraintForceX=off  SenseConstraintForceY=off  SenseConstraintForceZ=off  SenseConstraintTorque=off  SenseConstraintTorqueX=off  SenseConstraintTorqueY=off  SenseConstraintTorqueZ=off  SenseTotalForce=off  SenseTotalForceX=off  SenseTotalForceY=off  SenseTotalForceZ=off  SenseTotalTorque=off  SenseTotalTorqueX=off  SenseTotalTorqueY=off  SenseTotalTorqueZ=off  CompositeWrenchDir=FollowerOnBase  CompositeWrenchFrame=BaseFrame  EquilibriumPosition=0  EquilibriumPositionUnits=rad  SpringStiffness=0  SpringStiffnessUnits=N*m/rad  DampingCoefficient=0  DampingCoefficientUnits=N*m/(rad/s)  TorqueActuationMode=InputTorque  MotionActuationMode=ComputedMotion  SensePosition=on  SenseVelocity=on  SenseAcceleration=on  SenseTorqueForce=on  PositionTargetSpecify=on  PositionTargetPriority=Low  PositionTargetValue=smiData.RevoluteJoint(4).Rz.Pos  PositionTargetValueUnits=deg  VelocityTargetSpecify=off  VelocityTargetPriority=High  VelocityTargetValue=0  VelocityTargetValueUnits=deg/s
  Conn3 : PMIOPort  Side=Left
  Torque4 : PMIOPort  Port=2  Side=Left
  q4 : PMIOPort  Port=3  Side=Right
  w4 : PMIOPort  Port=4  Side=Right
  b4 : PMIOPort  Port=5  Side=Right
  t4 : PMIOPort  Port=6  Side=Right
  Conn4 : PMIOPort  Port=7  Side=Right
  connections:
  Torque4/RConn1 -- Revolute3/LConn2
  Link3_1_RIGID/RConn1 -- Revolute3/LConn1
  Link3_1_RIGID/LConn1 -- Conn3/RConn1
  PS Subtract1/LConn1 -- Revolute3/RConn2
  PS Subtract1/RConn1 -- q4/RConn1
  PS Constant2/RConn1 -- PS Subtract1/LConn2
  Conn4/RConn1 -- Revolute3/RConn1
  w4/RConn1 -- Revolute3/RConn3
  b4/RConn1 -- Revolute3/RConn4
  t4/RConn1 -- Revolute3/RConn5

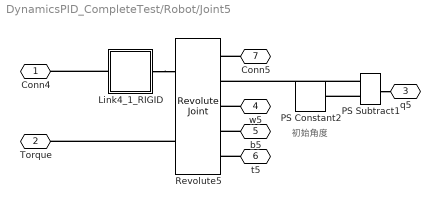
== system DynamicsPID_CompleteTest/Robot/Joint5 ==
  note: 初始角度
  Link4_1_RIGID : Subsystem
  PS Constant2 : fl_lib/Physical Signals/Sources/PS Constant  constant=pi/2
  PS Subtract1 : fl_lib/Physical Signals/Functions/PS Subtract
      settings: SourceProductName=Simscape
  Revolute5 : sm_lib/Joints/Revolute Joint  SenseConstraintForce=off  SenseConstraintForceX=off  SenseConstraintForceY=off  SenseConstraintForceZ=off  SenseConstraintTorque=off  SenseConstraintTorqueX=off  SenseConstraintTorqueY=off  SenseConstraintTorqueZ=off  SenseTotalForce=off  SenseTotalForceX=off  SenseTotalForceY=off  SenseTotalForceZ=off  SenseTotalTorque=off  SenseTotalTorqueX=off  SenseTotalTorqueY=off  SenseTotalTorqueZ=off  CompositeWrenchDir=FollowerOnBase  CompositeWrenchFrame=BaseFrame  EquilibriumPosition=0  EquilibriumPositionUnits=rad  SpringStiffness=0  SpringStiffnessUnits=N*m/rad  DampingCoefficient=0  DampingCoefficientUnits=N*m/(rad/s)  TorqueActuationMode=InputTorque  MotionActuationMode=ComputedMotion  SensePosition=on  SenseVelocity=on  SenseAcceleration=on  SenseTorqueForce=on  PositionTargetSpecify=on  PositionTargetPriority=Low  PositionTargetValue=smiData.RevoluteJoint(5).Rz.Pos  PositionTargetValueUnits=deg  VelocityTargetSpecify=off  VelocityTargetPriority=High  VelocityTargetValue=0  VelocityTargetValueUnits=deg/s
  Conn4 : PMIOPort  Side=Left
  Torque : PMIOPort  Port=2  Side=Left
  q5 : PMIOPort  Port=3  Side=Right
  w5 : PMIOPort  Port=4  Side=Right
  b5 : PMIOPort  Port=5  Side=Right
  t5 : PMIOPort  Port=6  Side=Right
  Conn5 : PMIOPort  Port=7  Side=Right
  connections:
  Link4_1_RIGID/RConn1 -- Revolute5/LConn1
  Revolute5/LConn2 -- Torque/RConn1
  Link4_1_RIGID/LConn1 -- Conn4/RConn1
  PS Subtract1/LConn1 -- Revolute5/RConn2
  PS Subtract1/RConn1 -- q5/RConn1
  PS Subtract1/LConn2 -- PS Constant2/RConn1
  Conn5/RConn1 -- Revolute5/RConn1
  w5/RConn1 -- Revolute5/RConn3
  b5/RConn1 -- Revolute5/RConn4
  t5/RConn1 -- Revolute5/RConn5

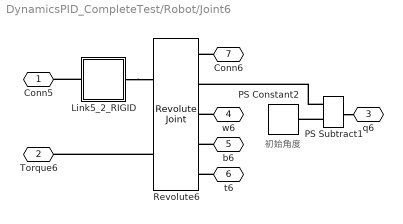
== system DynamicsPID_CompleteTest/Robot/Joint6 ==
  note: 初始角度
  Link5_2_RIGID : Subsystem
  PS Constant2 : fl_lib/Physical Signals/Sources/PS Constant  constant=-pi
  PS Subtract1 : fl_lib/Physical Signals/Functions/PS Subtract
      settings: SourceProductName=Simscape
  Revolute6 : sm_lib/Joints/Revolute Joint  SenseConstraintForce=off  SenseConstraintForceX=off  SenseConstraintForceY=off  SenseConstraintForceZ=off  SenseConstraintTorque=off  SenseConstraintTorqueX=off  SenseConstraintTorqueY=off  SenseConstraintTorqueZ=off  SenseTotalForce=off  SenseTotalForceX=off  SenseTotalForceY=off  SenseTotalForceZ=off  SenseTotalTorque=off  SenseTotalTorqueX=off  SenseTotalTorqueY=off  SenseTotalTorqueZ=off  CompositeWrenchDir=FollowerOnBase  CompositeWrenchFrame=BaseFrame  EquilibriumPosition=0  EquilibriumPositionUnits=rad  SpringStiffness=0  SpringStiffnessUnits=N*m/rad  DampingCoefficient=0  DampingCoefficientUnits=N*m/(rad/s)  TorqueActuationMode=InputTorque  MotionActuationMode=ComputedMotion  SensePosition=on  SenseVelocity=on  SenseAcceleration=on  SenseTorqueForce=on  PositionTargetSpecify=on  PositionTargetPriority=Low  PositionTargetValue=smiData.RevoluteJoint(6).Rz.Pos  PositionTargetValueUnits=deg  VelocityTargetSpecify=off  VelocityTargetPriority=High  VelocityTargetValue=0  VelocityTargetValueUnits=deg/s
  Conn5 : PMIOPort  Side=Left
  Torque6 : PMIOPort  Port=2  Side=Left
  q6 : PMIOPort  Port=3  Side=Right
  w6 : PMIOPort  Port=4  Side=Right
  b6 : PMIOPort  Port=5  Side=Right
  t6 : PMIOPort  Port=6  Side=Right
  Conn6 : PMIOPort  Port=7  Side=Right
  connections:
  Link5_2_RIGID/RConn1 -- Revolute6/LConn1
  Link5_2_RIGID/LConn1 -- Conn5/RConn1
  PS Subtract1/LConn1 -- Revolute6/RConn2
  Revolute6/LConn2 -- Torque6/RConn1
  PS Subtract1/RConn1 -- q6/RConn1
  PS Subtract1/LConn2 -- PS Constant2/RConn1
  Conn6/RConn1 -- Revolute6/RConn1
  w6/RConn1 -- Revolute6/RConn3
  b6/RConn1 -- Revolute6/RConn4
  t6/RConn1 -- Revolute6/RConn5

== system DynamicsPID_CompleteTest/Robot/Link6_1_RIGID ==
  ReferenceFrame : sm_lib/Frames and Transforms/Reference Frame
  Solid : sm_lib/Body Elements/Solid  InertiaType=Custom  Mass=smiData.Solid(6).mass  MassUnits=kg  CenterOfMass=smiData.Solid(6).CoM  CenterOfMassUnits=mm  MomentsOfInertia=smiData.Solid(6).MoI  MomentsOfInertiaUnits=kg*mm^2  ProductsOfInertia=smiData.Solid(6).PoI  ProductsOfInertiaUnits=kg*mm^2  BasedOnType=DensityFromFile  Density=1000  DensityUnits=kg/m^3  DoExposeReferenceFrame=on  SerializedFrames=<Frames/>  GraphicType=FromGeometry  MarkerShape=Sphere  MarkerSize=10  GraphicVisPropType=SimpleVisualProperties  GraphicDiffuseColor=smiData.Solid(6).color  GraphicSpecularColor=[0.5 0.5 0.5 1.0]  GraphicAmbientColor=[0.15 0.15 0.15 1.0]  GraphicEmissiveColor=[0.0 0.0 0.0 1.0]  GraphicShininess=75  GraphicOpacity=smiData.Solid(6).opacity  GeometryShape=FromFile  RectangleSize=[1 1]  RectangleSizeUnits=m  BrickDimensions=[1 1 1]  BrickDimensionUnits=m  CylinderRadius=1  CylinderRadiusUnits=m  CylinderLength=1  CylinderLengthUnits=m  SphereRadius=1  SphereRadiusUnits=m  EllipsoidRadii=[1 1 1]  EllipsoidRadiiUnits=m  ExtrusionCrossSection=[1 1; -1 1; -1 -1; 1 -1]  ExtrusionCrossSectionUnits=m  ExtrusionLength=1  ExtrusionLengthUnits=m  PolygonNumSides=3  PolygonOuterRadius=1  PolygonOuterRadiusUnits=m  ExtGeomFileType=STEP  ExtGeomFileName=Link6_默认_sldprt.STEP  ExtGeomFileUnits=m  RevolutionCrossSection=[1 1; 1 -1; 2 -1; 2 1]  RevolutionCrossSectionUnits=m  RevolutionExtent=Full  RevolutionAngle=180  RevolutionAngleUnits=deg
  Transform : sm_lib/Frames and Transforms/Rigid Transform  TranslationMethod=Cartesian  TranslationStandardOffset=0  TranslationLengthUnit=mm  TranslationStandardAxis=+Z  TranslationCartesianOffset=smiData.RigidTransform(12).translation  TranslationROffset=0  TranslationROffsetUnits=m  TranslationZOffset=0  TranslationZOffsetUnits=m  TranslationThetaOffset=0  TranslationThetaOffsetUnits=deg  RotationMethod=ArbitraryAxis  RotationAngleUnits=rad  RotationStandardAxis=+Z  RotationAngle=smiData.RigidTransform(12).angle  RotationArbitraryAxis=smiData.RigidTransform(12).axis  FollAlignAxisA=+X  BaseAlignAxisA=+Y  FollAlignAxisB=+Y  BaseAlignAxisB=+Z  RotationSequenceAxes=FollowerAxes  RotationSequence=XYX  RotationSequenceAngles=[0 0 0]  RotationSequenceAnglesUnits=deg  RotationMatrix=[1 0 0; 0 1 0; 0 0 1]
  F : PMIOPort  Side=Left
  connections:
  Solid/RConn1 -- ReferenceFrame/RConn1 -- Transform/LConn1
  Transform/RConn1 -- F/RConn1

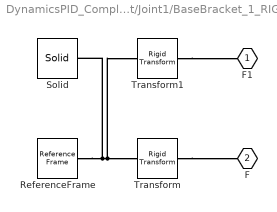
== system DynamicsPID_CompleteTest/Robot/Joint1/BaseBracket_1_RIGID ==
  ReferenceFrame : sm_lib/Frames and Transforms/Reference Frame
  Solid : sm_lib/Body Elements/Solid  InertiaType=Custom  Mass=smiData.Solid(7).mass  MassUnits=kg  CenterOfMass=smiData.Solid(7).CoM  CenterOfMassUnits=mm  MomentsOfInertia=smiData.Solid(7).MoI  MomentsOfInertiaUnits=kg*mm^2  ProductsOfInertia=smiData.Solid(7).PoI  ProductsOfInertiaUnits=kg*mm^2  BasedOnType=DensityFromFile  Density=1000  DensityUnits=kg/m^3  DoExposeReferenceFrame=on  SerializedFrames=<Frames/>  GraphicType=FromGeometry  MarkerShape=Sphere  MarkerSize=10  GraphicVisPropType=SimpleVisualProperties  GraphicDiffuseColor=smiData.Solid(7).color  GraphicSpecularColor=[0.5 0.5 0.5 1.0]  GraphicAmbientColor=[0.15 0.15 0.15 1.0]  GraphicEmissiveColor=[0.0 0.0 0.0 1.0]  GraphicShininess=75  GraphicOpacity=smiData.Solid(7).opacity  GeometryShape=FromFile  RectangleSize=[1 1]  RectangleSizeUnits=m  BrickDimensions=[1 1 1]  BrickDimensionUnits=m  CylinderRadius=1  CylinderRadiusUnits=m  CylinderLength=1  CylinderLengthUnits=m  SphereRadius=1  SphereRadiusUnits=m  EllipsoidRadii=[1 1 1]  EllipsoidRadiiUnits=m  ExtrusionCrossSection=[1 1; -1 1; -1 -1; 1 -1]  ExtrusionCrossSectionUnits=m  ExtrusionLength=1  ExtrusionLengthUnits=m  PolygonNumSides=3  PolygonOuterRadius=1  PolygonOuterRadiusUnits=m  ExtGeomFileType=STEP  ExtGeomFileName=BaseBracket_默认_sldprt.STEP  ExtGeomFileUnits=m  RevolutionCrossSection=[1 1; 1 -1; 2 -1; 2 1]  RevolutionCrossSectionUnits=m  RevolutionExtent=Full  RevolutionAngle=180  RevolutionAngleUnits=deg
  Transform : sm_lib/Frames and Transforms/Rigid Transform  TranslationMethod=Cartesian  TranslationStandardOffset=0  TranslationLengthUnit=mm  TranslationStandardAxis=+Z  TranslationCartesianOffset=smiData.RigidTransform(3).translation  TranslationROffset=0  TranslationROffsetUnits=m  TranslationZOffset=0  TranslationZOffsetUnits=m  TranslationThetaOffset=0  TranslationThetaOffsetUnits=deg  RotationMethod=ArbitraryAxis  RotationAngleUnits=rad  RotationStandardAxis=+Z  RotationAngle=smiData.RigidTransform(3).angle  RotationArbitraryAxis=smiData.RigidTransform(3).axis  FollAlignAxisA=+X  BaseAlignAxisA=+Y  FollAlignAxisB=+Y  BaseAlignAxisB=+Z  RotationSequenceAxes=FollowerAxes  RotationSequence=XYX  RotationSequenceAngles=[0 0 0]  RotationSequenceAnglesUnits=deg  RotationMatrix=[1 0 0; 0 1 0; 0 0 1]
  Transform1 : sm_lib/Frames and Transforms/Rigid Transform  TranslationMethod=Cartesian  TranslationStandardOffset=0  TranslationLengthUnit=mm  TranslationStandardAxis=+Z  TranslationCartesianOffset=smiData.RigidTransform(13).translation  TranslationROffset=0  TranslationROffsetUnits=m  TranslationZOffset=0  TranslationZOffsetUnits=m  TranslationThetaOffset=0  TranslationThetaOffsetUnits=deg  RotationMethod=ArbitraryAxis  RotationAngleUnits=rad  RotationStandardAxis=+Z  RotationAngle=smiData.RigidTransform(13).angle  RotationArbitraryAxis=smiData.RigidTransform(13).axis  FollAlignAxisA=+X  BaseAlignAxisA=+Y  FollAlignAxisB=+Y  BaseAlignAxisB=+Z  RotationSequenceAxes=FollowerAxes  RotationSequence=XYX  RotationSequenceAngles=[0 0 0]  RotationSequenceAnglesUnits=deg  RotationMatrix=[1 0 0; 0 1 0; 0 0 1]
  F1 : PMIOPort  Side=Left
  F : PMIOPort  Port=2  Side=Right
  connections:
  Solid/RConn1 -- ReferenceFrame/RConn1 -- Transform/LConn1 -- Transform1/LConn1
  Transform/RConn1 -- F/RConn1
  Transform1/RConn1 -- F1/RConn1

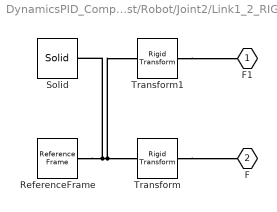
== system DynamicsPID_CompleteTest/Robot/Joint2/Link1_2_RIGID ==
  ReferenceFrame : sm_lib/Frames and Transforms/Reference Frame
  Solid : sm_lib/Body Elements/Solid  InertiaType=Custom  Mass=smiData.Solid(3).mass  MassUnits=kg  CenterOfMass=smiData.Solid(3).CoM  CenterOfMassUnits=mm  MomentsOfInertia=smiData.Solid(3).MoI  MomentsOfInertiaUnits=kg*mm^2  ProductsOfInertia=smiData.Solid(3).PoI  ProductsOfInertiaUnits=kg*mm^2  BasedOnType=DensityFromFile  Density=1000  DensityUnits=kg/m^3  DoExposeReferenceFrame=on  SerializedFrames=<Frames/>  GraphicType=FromGeometry  MarkerShape=Sphere  MarkerSize=10  GraphicVisPropType=SimpleVisualProperties  GraphicDiffuseColor=smiData.Solid(3).color  GraphicSpecularColor=[0.5 0.5 0.5 1.0]  GraphicAmbientColor=[0.15 0.15 0.15 1.0]  GraphicEmissiveColor=[0.0 0.0 0.0 1.0]  GraphicShininess=75  GraphicOpacity=smiData.Solid(3).opacity  GeometryShape=FromFile  RectangleSize=[1 1]  RectangleSizeUnits=m  BrickDimensions=[1 1 1]  BrickDimensionUnits=m  CylinderRadius=1  CylinderRadiusUnits=m  CylinderLength=1  CylinderLengthUnits=m  SphereRadius=1  SphereRadiusUnits=m  EllipsoidRadii=[1 1 1]  EllipsoidRadiiUnits=m  ExtrusionCrossSection=[1 1; -1 1; -1 -1; 1 -1]  ExtrusionCrossSectionUnits=m  ExtrusionLength=1  ExtrusionLengthUnits=m  PolygonNumSides=3  PolygonOuterRadius=1  PolygonOuterRadiusUnits=m  ExtGeomFileType=STEP  ExtGeomFileName=Link1_默认_sldprt.STEP  ExtGeomFileUnits=m  RevolutionCrossSection=[1 1; 1 -1; 2 -1; 2 1]  RevolutionCrossSectionUnits=m  RevolutionExtent=Full  RevolutionAngle=180  RevolutionAngleUnits=deg
  Transform : sm_lib/Frames and Transforms/Rigid Transform  TranslationMethod=Cartesian  TranslationStandardOffset=0  TranslationLengthUnit=mm  TranslationStandardAxis=+Z  TranslationCartesianOffset=smiData.RigidTransform(1).translation  TranslationROffset=0  TranslationROffsetUnits=m  TranslationZOffset=0  TranslationZOffsetUnits=m  TranslationThetaOffset=0  TranslationThetaOffsetUnits=deg  RotationMethod=ArbitraryAxis  RotationAngleUnits=rad  RotationStandardAxis=+Z  RotationAngle=smiData.RigidTransform(1).angle  RotationArbitraryAxis=smiData.RigidTransform(1).axis  FollAlignAxisA=+X  BaseAlignAxisA=+Y  FollAlignAxisB=+Y  BaseAlignAxisB=+Z  RotationSequenceAxes=FollowerAxes  RotationSequence=XYX  RotationSequenceAngles=[0 0 0]  RotationSequenceAnglesUnits=deg  RotationMatrix=[1 0 0; 0 1 0; 0 0 1]
  Transform1 : sm_lib/Frames and Transforms/Rigid Transform  TranslationMethod=Cartesian  TranslationStandardOffset=0  TranslationLengthUnit=mm  TranslationStandardAxis=+Z  TranslationCartesianOffset=smiData.RigidTransform(4).translation  TranslationROffset=0  TranslationROffsetUnits=m  TranslationZOffset=0  TranslationZOffsetUnits=m  TranslationThetaOffset=0  TranslationThetaOffsetUnits=deg  RotationMethod=ArbitraryAxis  RotationAngleUnits=rad  RotationStandardAxis=+Z  RotationAngle=smiData.RigidTransform(4).angle  RotationArbitraryAxis=smiData.RigidTransform(4).axis  FollAlignAxisA=+X  BaseAlignAxisA=+Y  FollAlignAxisB=+Y  BaseAlignAxisB=+Z  RotationSequenceAxes=FollowerAxes  RotationSequence=XYX  RotationSequenceAngles=[0 0 0]  RotationSequenceAnglesUnits=deg  RotationMatrix=[1 0 0; 0 1 0; 0 0 1]
  F1 : PMIOPort  Side=Left
  F : PMIOPort  Port=2  Side=Right
  connections:
  Solid/RConn1 -- ReferenceFrame/RConn1 -- Transform/LConn1 -- Transform1/LConn1
  Transform/RConn1 -- F/RConn1
  Transform1/RConn1 -- F1/RConn1
